simulink model "quadSimulationEnvironment"  (R2022b)
settings: Solver=ode4  StartTime=0.0  StopTime=20  FixedStep=.005  RelTol=1e-3  EnableMultiTasking=on
InitFcn:
  | %%General
  | dT = .005;
  | m = .68;
  | g = 9.8;
  | mg = m*g;
  | 
  | s = tf('s');
  | %%Servomotors
  | h_alpha = 200;
  | 
  | servo_limit = 2500;
  | servo_ratelimit = 450*pi/180/1.33e-4;
  | servo_sampleDelay = 1;
  | servo_wn = 28;
  | servo_zeta = .6;
  | servo_dtime = 5e-3;
  | servo_res = 10;
  | servo_sf = 1/6700;
  | %motor
  | motor_w = 20;
  | motor_dtime = 5e-3;
  | motor_wo = 600;
  | %%Rotors
  | Pw_v = .244/(1+s*.287);
  | Pw_a = -.10/(1+s*.30)*eye(4,4);
  | 
  | motor_limit = 13107;
  | %%Speed control
  | xw = .102/.234;
  | Xw = xw*eye(4,4);
  | 
  | fw = 1/(1+s/1);
  | Fw = fw*eye(4,4);
  | Fw = c2d(Fw,.005,'tustin');
  | 
  | gw = 12.77*(1+s/4)/s/(1+s/21);
  | Gw = gw*eye(4,4);
  | Gw = c2d(Gw,.005,'tustin');
  | %%Thrust control
  | gf = 10628*(1+s/26)*(1+s/44)/s/(1+s/247);
  | Gf = gf*eye(4,4);
  | Gf = c2d(Gf,.005,'tustin');
  | 
  | xf = 358/( s^2/21^2+2*.38/21*s+1);
  | Xf = xf*eye(4,4);
  | Xf = c2d(Xf,.005,'tustin');
  | 
  | %%Attitude control
  | gxy = 7.77*(s+.6443)/(s+268.4);
  | gz = .062*(1+s/3.37)/s/(1+s/169);
  | Gn = [gxy 0 0;
  |       0 gxy 0;
  |       0 0 gz];
  | Gn = c2d(Gn,.005,'tustin');
  | 
  | %%Position control
  | % gp = 151.34*(s+1.925)/(s+81.18);
  | gp = 117.96*(s+0.5)*(s+0.7839)/s/(s+71.75);
  | Gp = gp*eye(3);
  | Gp = c2d(Gp,.005,'tustin');
  | 
  | wp = 4;
  | zp = 1.0;
  | fp = wp^2/(s^2+2*zp*wp*s+wp^2);
  | Fp = fp*eye(3);
  | Fp = c2d(Fp,.005,'tustin');
  | 
  | xp = -.34*(1+s/.5)/(1+s/25.57)*(1+s/11.93)/(1+s/21.7);
  | Xp = xp*eye(3);
  | Xp = c2d(Xp,.005,'tustin');
undefined symbols (not defined in the file or in its folder): Kp, pl_wn, pl_z, w_der, wf_p1, wf_p2, wf_z1, wf_z2, wmr, wp_p, wp_z, wp_z2, wt, zmr, zt
libraries: cstblocks x14, simulink_extras x6, simulink x5, sharedutil x5, uavutilslib x1, matrix_library x1, aerolibutil x1
settings Model: Creator=Arnold  LastModifiedBy=arnoldpretorius
settings SolverCC: AlgebraicLoopSolver=TrustRegion
settings DataIOCC: LimitDataPoints=on  SaveFormat=Array  ReturnWorkspaceOutputs=off
settings OptimizationCC: ExpressionDepthLimit=2147483647  LifeSpan=inf
settings DebuggingCC: UnderspecifiedInitializationDetection=Classic  MergeDetectMultiDrivingBlocksExec=none  SolverPrmCheckMsg=warning  UnconnectedInputMsg=warning  UnconnectedOutputMsg=warning  UnconnectedLineMsg=warning  StateNameClashWarn=warning  SFUnexpectedBacktrackingDiag=warning  SFNoUnconditionalDefaultTransitionDiag=warning  SFExecutionAtInitializationDiag=none  SFMachineParentedDataDiag=warning  ArithmeticOperatorsInVariantConditions=warning
settings HardwareCC: ProdBitPerPointer=32  ProdBitPerSizeT=32  ProdBitPerPtrDiffT=32  ProdLargestAtomicFloat=None  ProdIntDivRoundTo=Undefined  ProdEndianess=Unspecified  ProdWordSize=32  ProdHWDeviceType=32-bit Generic
settings ModelReferenceCC: EnableRefExpFcnMdlSchedulingChecks=on  PropagateSignalLabelsOutOfModel=off
settings SFSimCC: SimUseLocalCustomCode=off  CustomCodeUndefinedFunction=UseInterfaceOnly
settings RTWCC: RTWUseLocalCustomCode=off  DLArmComputeVersion=19.05
settings CodeAppCC: StateflowObjectComments=on
settings GRTTargetCC: TargetLangStandard=C89/C90 (ANSI)
settings ConfigComp: CovMetricSettings=dw  CovSaveCumulativeToWorkspaceVar=on  CovSaveSingleToWorkspaceVar=on  CovExternalEMLEnable=off

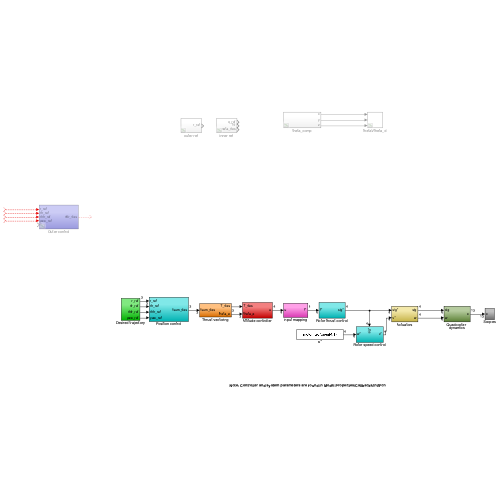
[thumbnail: Simulink's stored preview of the top-level diagram]
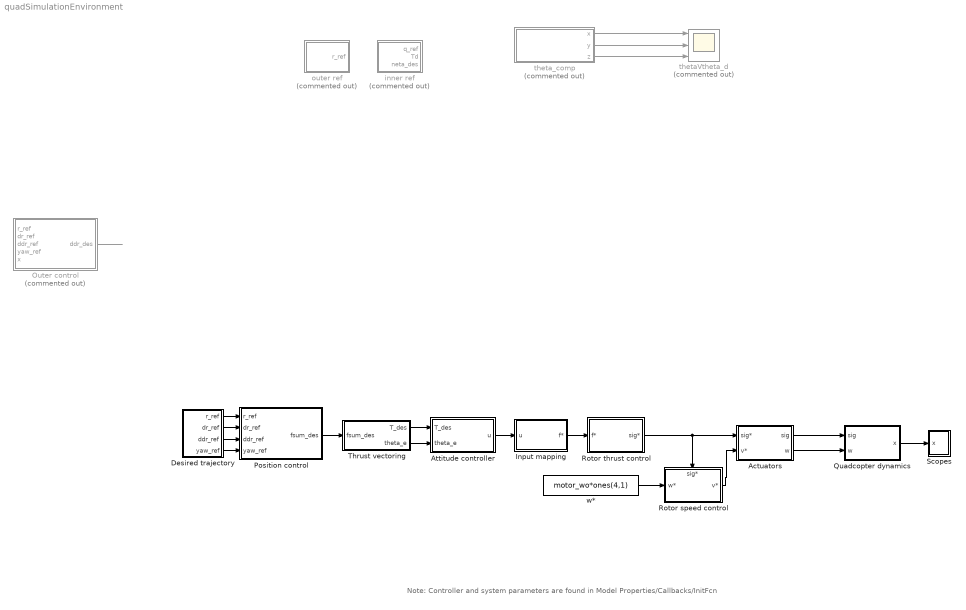
== system quadSimulationEnvironment ==
  note: Note: Controller and system parameters are found in Model Properties/Callbacks/InitFcn
  Actuators : Subsystem
  Attitude controller : Subsystem
  Desired trajectory : Subsystem
  Input mapping : Subsystem
  Outer control : Subsystem  Commented=on
  Position control : Subsystem
  Quadcopter dynamics : Subsystem
  Rotor speed control : Subsystem
      settings: PortSchema="{\"entries\":[{\"content\":{\"sides\":[{\"content\":{\"connectorIds\":[\"In1\"]},\"type\":\"ConnectorPlacement.EquallySpacedRectSide\",\"uuid\":\"a553ec9c-58d4-4b9a-a914-c6161034d4ac\"},{\"content\":{\"connectorIds\":[\"Out1\"],\"side\":\"RIGHT\"},\"type\":\"ConnectorPlacement.EquallySpacedRectSide\",\"uuid\":\"56d1cb9b-318c-4753-8a79-3897c75d4c58\"},{\"content\":{\"connectorIds\":[\"In2\"],\"side\":\"TOP\"},\"type\":\"ConnectorPlacement.EquallySpacedRectSide\",\"uuid\":\"ddf4192e-7ef8-4e19-bd18-fba4d537495f\"}]},\"type\":\"ConnectorPlacement.EquallySpacedConnector\",\"uuid\":\"ae11febd-5c1c-44f7-8744-831945371bf2\"}],\"packageUris\":[\"http://schema.mathworks.com/mf0/Connector/R2020b\"],\"version\":\"1.0\"}"
  Rotor thrust control : Subsystem
  Scopes : Subsystem
  Thrust vectoring : Subsystem
  inner ref : Subsystem  Commented=on
  outer ref : Subsystem  Commented=on
  thetaVtheta_d : Scope  Commented=on  NumInputPorts=3
  theta_comp : Subsystem  Commented=on
  w* : Constant  Value=motor_wo*ones(4,1)
  wires:
  Quadcopter dynamics/1(x) -> Scopes/1(x)
  Outer control/1(ddr_des) -> ?
  Actuators/1(sig) -> Quadcopter dynamics/1(sig)
  Actuators/2(w) -> Quadcopter dynamics/2(w)
  ? -> Outer control/1(r_ref)
  ? -> Outer control/2(dr_ref)
  ? -> Outer control/3(ddr_ref)
  ? -> Outer control/4(yaw_ref)
  Rotor thrust control/1(sig*) -> Actuators/1(sig*), Rotor speed control/2(sig*)
  Rotor speed control/1(v*) -> Actuators/2(v*)
  Input mapping/1(f*) -> Rotor thrust control/1(f*)
  Attitude controller/1(u) -> Input mapping/1(u)
  Thrust vectoring/1(T_des) -> Attitude controller/1(T_des)
  Thrust vectoring/2(theta_e) -> Attitude controller/2(theta_e)
  theta_comp/1(x) -> thetaVtheta_d/1
  theta_comp/3(z) -> thetaVtheta_d/3
  theta_comp/2(y) -> thetaVtheta_d/2
  Position control/1(fsum_des) -> Thrust vectoring/1(fsum_des)
  Desired trajectory/2(dr_ref) -> Position control/2(dr_ref)
  Desired trajectory/4(yaw_ref) -> Position control/4(yaw_ref)
  Desired trajectory/1(r_ref) -> Position control/1(r_ref)
  Desired trajectory/3(ddr_ref) -> Position control/3(ddr_ref)
  w*/1 -> Rotor speed control/1(w*)

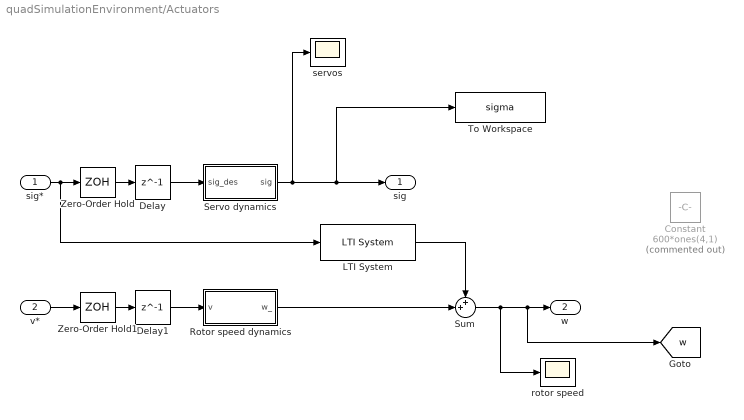
== system quadSimulationEnvironment/Actuators ==
  sig* : Inport
  v* : Inport  Port=2
  Constant : Constant  Commented=on  Value=600*ones(4,1)
  Delay : Delay  DelayLength=1  SampleTime=dT
  Delay1 : Delay  DelayLength=1  SampleTime=dT
  LTI System : cstblocks/LTI System  sys=Pw_a  IC=[]
  Rotor speed dynamics : Subsystem
  Servo dynamics : Subsystem
  Sum : Sum  Inputs=++|
  To Workspace : ToWorkspace  VariableName=sigma  SaveFormat=Timeseries  SampleTime=-1
  Zero-Order Hold : ZeroOrderHold  SampleTime=servo_dtime
  Zero-Order Hold1 : ZeroOrderHold  SampleTime=motor_dtime
  rotor speed : Scope
  servos : Scope
  sig : Outport
  w : Outport  Port=2
  tag scope: w=global
  wires:
  Servo dynamics/1(sig) -> servos/1, To Workspace/1, sig/1
  sig*/1 -> LTI System/1, Zero-Order Hold/1
  v*/1 -> Zero-Order Hold1/1
  Delay1/1 -> Rotor speed dynamics/1(v)
  Delay/1 -> Servo dynamics/1(sig_des)
  Zero-Order Hold/1 -> Delay/1
  Zero-Order Hold1/1 -> Delay1/1
  Sum/1 -> rotor speed/1, [w], w/1
  Rotor speed dynamics/1(w_) -> Sum/2
  LTI System/1 -> Sum/1

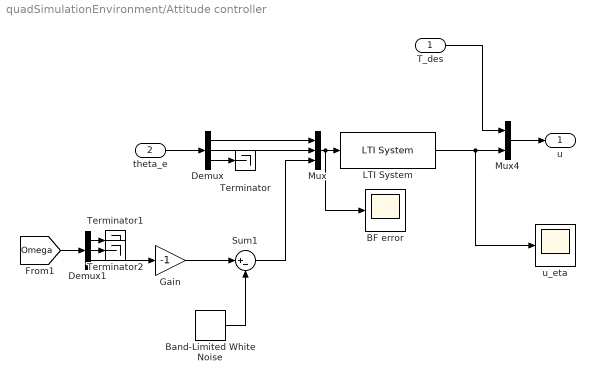
== system quadSimulationEnvironment/Attitude controller ==
  T_des : Inport
  theta_e : Inport  Port=2
  BF error : Scope
  Band-Limited White Noise : simulink/Sources/Band-Limited White Noise  Cov=[0.0004]  Ts=0.005  seed=[123]
  Demux : Demux  Outputs=3
  Demux1 : Demux  Outputs=3
  Gain : Gain  Gain=-1
  LTI System : cstblocks/LTI System  sys=Gn  IC=[]
  Mux : Mux  Inputs=3
  Mux4 : Mux  Inputs=2
  Sum1 : Sum  Inputs=|+-
  Terminator : Terminator
  Terminator1 : Terminator
  Terminator2 : Terminator
  u_eta : Scope
  u : Outport
  wires:
  LTI System/1 -> u_eta/1, Mux4/2
  Mux4/1 -> u/1
  T_des/1 -> Mux4/1
  theta_e/1 -> Demux/1
  Mux/1 -> BF error/1, LTI System/1
  Demux/1 -> Mux/1
  Demux/2 -> Mux/2
  Demux/3 -> Terminator/1
  [Omega] -> Demux1/1
  Demux1/3 -> Gain/1
  Demux1/1 -> Terminator1/1
  Demux1/2 -> Terminator2/1
  Gain/1 -> Sum1/1
  Sum1/1 -> Mux/3
  Band-Limited White Noise/1 -> Sum1/2

== system quadSimulationEnvironment/Desired trajectory ==
  Gain : Gain  Gain=-1
  LTI System : cstblocks/LTI System  sys=fp  IC=[]
  LTI System1 : cstblocks/LTI System  sys=fp  IC=[]
  Mux1 : Mux  Inputs=3
  Step1 : Step  Time=10  SampleTime=0
  Step2 : Step  Time=3  SampleTime=0
  r_ref : Outport
  dr_ref : Outport  Port=2
  ddr_ref : Outport  Port=3
  yaw_ref : Outport  Port=4
  wires:
  Mux1/1 -> r_ref/1
  Step1/1 -> LTI System/1
  Gain/1 -> Mux1/2
  Step2/1 -> LTI System1/1
  LTI System/1 -> Gain/1, Mux1/1
  LTI System1/1 -> Mux1/3

== system quadSimulationEnvironment/Input mapping ==
  u : Inport
  Display1 : Display
  Display2 : Display
  "input2sig_des " : MATLAB Function  TreatAsAtomicUnit=on
  mixing : MATLAB Function  Commented=on  TreatAsAtomicUnit=on
  yawFreeSig : MATLAB Function  Commented=on  TreatAsAtomicUnit=on
  f* : Outport
  wires:
  u/1 -> "input2sig_des "/1(u)
  "input2sig_des "/1(f_des) -> Display1/1, f*/1

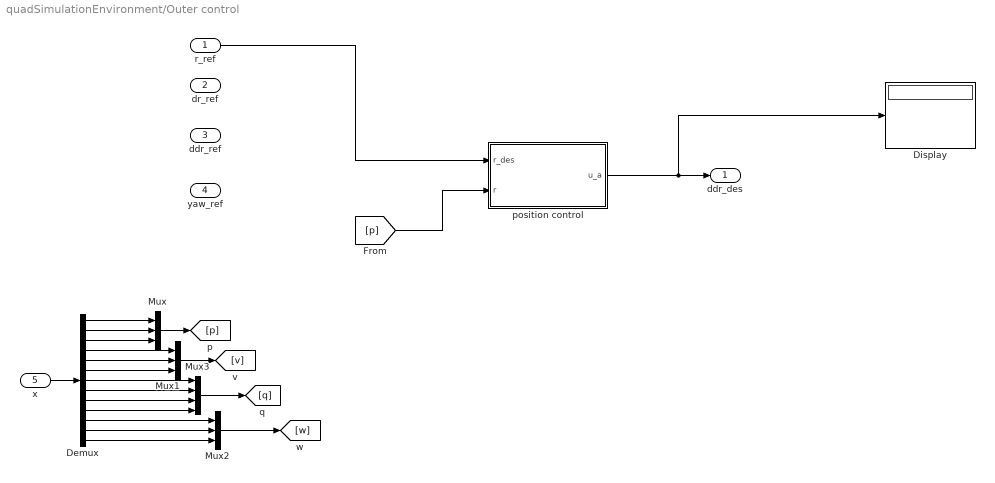
== system quadSimulationEnvironment/Outer control ==
  r_ref : Inport
  dr_ref : Inport  Port=2
  ddr_ref : Inport  Port=3
  yaw_ref : Inport  Port=4
  x : Inport  Port=5
  Demux : Demux  Outputs=13
  Display : Display
  Mux : Mux  Inputs=3
  Mux1 : Mux  Inputs=3
  Mux2 : Mux  Inputs=3
  Mux3 : Mux
  position control : Subsystem
  ddr_des : Outport
  wires:
  r_ref/1 -> position control/1(r_des)
  [p] -> position control/2(r)
  position control/1(u_a) -> Display/1, ddr_des/1
  x/1 -> Demux/1
  Demux/1 -> Mux/1
  Demux/2 -> Mux/2
  Demux/3 -> Mux/3
  Demux/4 -> Mux1/1
  Demux/5 -> Mux1/2
  Demux/6 -> Mux1/3
  Demux/7 -> Mux3/1
  Demux/8 -> Mux3/2
  Demux/9 -> Mux3/3
  Mux1/1 -> [v]
  Mux/1 -> [p]
  Demux/10 -> Mux3/4
  Demux/11 -> Mux2/1
  Demux/12 -> Mux2/2
  Demux/13 -> Mux2/3
  Mux3/1 -> [q]
  Mux2/1 -> [w]

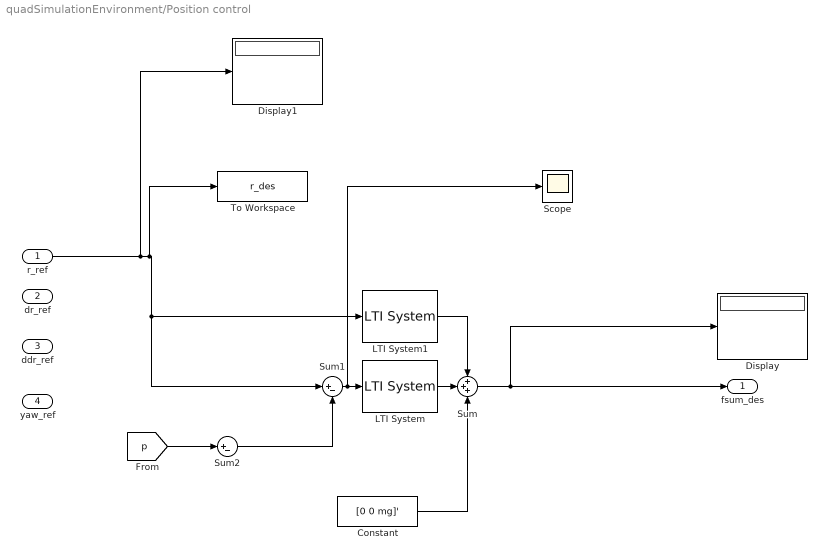
== system quadSimulationEnvironment/Position control ==
  r_ref : Inport
  dr_ref : Inport  Port=2
  ddr_ref : Inport  Port=3
  yaw_ref : Inport  Port=4
  Constant : Constant  Value=[0 0 mg]'
  Display : Display
  Display1 : Display
  LTI System : cstblocks/LTI System  sys=Gp  IC=[]
  LTI System1 : cstblocks/LTI System  sys=Xp  IC=[]
  Scope : Scope
  Sum : Sum  Inputs=+++
  Sum1 : Sum  Inputs=|+-
  Sum2 : Sum  Inputs=|+-
  To Workspace : ToWorkspace  VariableName=r_des  SaveFormat=Timeseries  SampleTime=-1
  fsum_des : Outport
  wires:
  r_ref/1 -> Display1/1, To Workspace/1, LTI System1/1, Sum1/1
  Sum/1 -> Display/1, fsum_des/1
  LTI System/1 -> Sum/2
  Constant/1 -> Sum/3
  Sum1/1 -> Scope/1, LTI System/1
  [p] -> Sum2/1
  Sum2/1 -> Sum1/2
  LTI System1/1 -> Sum/1

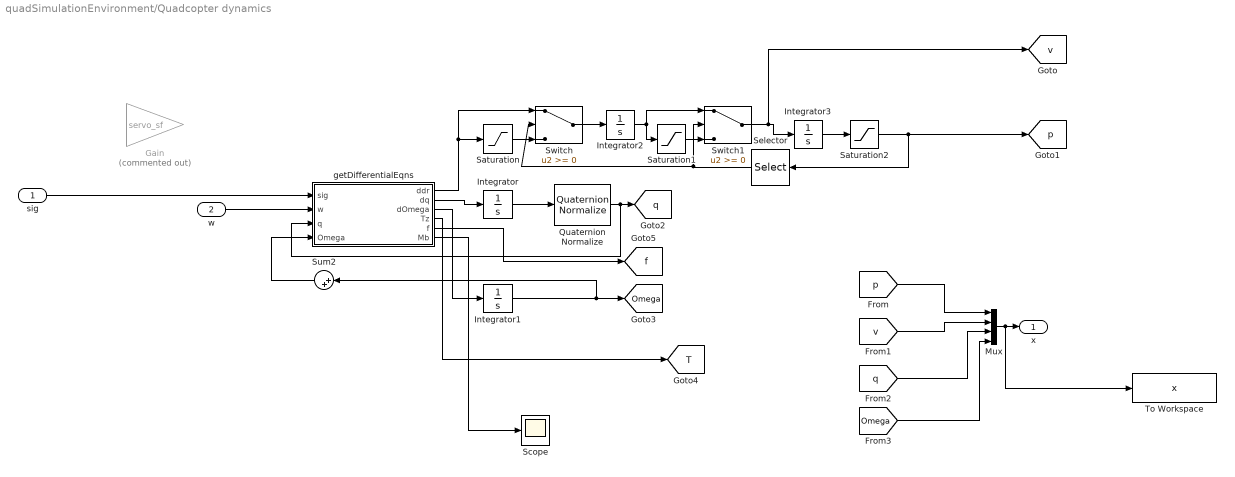
== system quadSimulationEnvironment/Quadcopter dynamics ==
  sig : Inport
  w : Inport  Port=2
  Gain : Gain  Commented=on  Gain=servo_sf
  Integrator : Integrator  InitialCondition=[1 0 0 0]
  Integrator1 : Integrator  InitialCondition=[0 0 0]
  Integrator2 : Integrator  InitialCondition=[0 0 0]
  Integrator3 : Integrator  InitialCondition=[0 0 0]
  Mux : Mux
  Quaternion Normalize : sharedutil/Quaternion Normalize  aMode=aMode
  Saturation : Saturate  UpperLimit=[1e10 1e10 1e10]  LowerLimit=[-1e10 -1e10 0]
  Saturation1 : Saturate  UpperLimit=[1e10 1e10 1e10]  LowerLimit=[-1e10 -1e10 0]
  Saturation2 : Saturate  UpperLimit=[1e10 1e10 1e10]  LowerLimit=[-1e10 -1e10 0]
  Scope : Scope
  Selector : Selector  InputPortWidth=3  IndexOptions=Index vector (dialog)  Indices=[3]  OutputSizes=1
  Sum2 : Sum  Inputs=|++
  Switch : Switch  SaturateOnIntegerOverflow=off  InputSameDT=off
  Switch1 : Switch  SaturateOnIntegerOverflow=off  InputSameDT=off
  To Workspace : ToWorkspace  VariableName=x  SaveFormat=Timeseries  SampleTime=-1
  getDifferentialEqns : MATLAB Function  TreatAsAtomicUnit=on
  x : Outport
  tag scope: Omega=global, T=global, f=global, p=global, q=global, v=global
  wires:
  w/1 -> getDifferentialEqns/2(w)
  getDifferentialEqns/2(dq) -> Integrator/1
  Integrator/1 -> Quaternion Normalize/1
  getDifferentialEqns/3(dOmega) -> Integrator1/1
  Integrator1/1 -> Sum2/1, [Omega]
  Integrator3/1 -> Saturation2/1
  Mux/1 -> To Workspace/1, x/1
  [p] -> Mux/1
  [v] -> Mux/2
  [q] -> Mux/3
  [Omega] -> Mux/4
  getDifferentialEqns/4(Tz) -> [T]
  getDifferentialEqns/5(f) -> [f]
  sig/1 -> getDifferentialEqns/1(sig)
  Quaternion Normalize/1 -> getDifferentialEqns/3(q), [q]
  getDifferentialEqns/6(Mb) -> Scope/1
  getDifferentialEqns/1(ddr) -> Saturation/1, Switch/1
  Sum2/1 -> getDifferentialEqns/4(Omega)
  Saturation/1 -> Switch/3
  Switch/1 -> Integrator2/1
  Integrator2/1 -> Saturation1/1, Switch1/1
  Saturation1/1 -> Switch1/3
  Switch1/1 -> [v], Integrator3/1
  Saturation2/1 -> Selector/1, [p]
  Selector/1 -> Switch1/2, Switch/2

== system quadSimulationEnvironment/Rotor speed control ==
  w* : Inport
  sig* : Inport  Port=2
  LTI System : cstblocks/LTI System  sys=Gw  IC=[]
  LTI System1 : cstblocks/LTI System  sys=Xw  IC=[]
  Sum : Sum  Inputs=|+-
  Sum1 : Sum  Inputs=++|
  v* : Outport
  wires:
  w*/1 -> Sum/1
  [w] -> Sum/2
  Sum/1 -> LTI System/1
  LTI System/1 -> Sum1/2
  LTI System1/1 -> Sum1/1
  Sum1/1 -> v*/1
  sig*/1 -> LTI System1/1

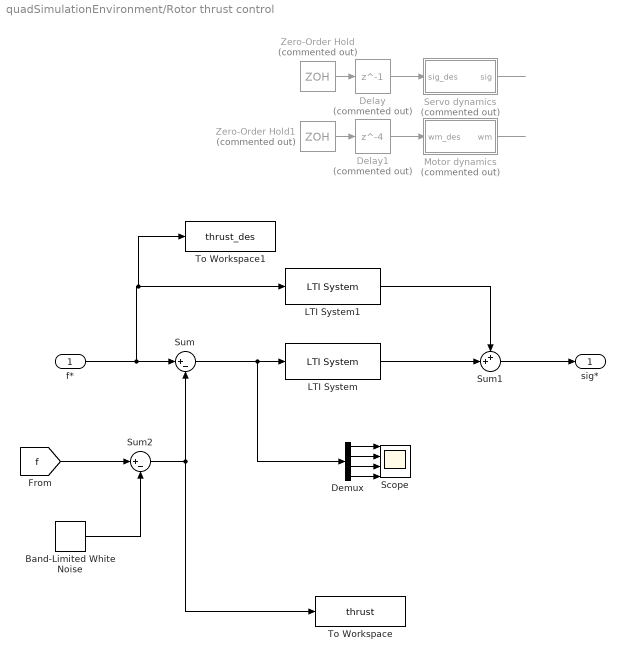
== system quadSimulationEnvironment/Rotor thrust control ==
  f* : Inport
  Band-Limited White Noise : simulink/Sources/Band-Limited White Noise  Cov=[0.000008]  Ts=0.005  seed=[23341]
  Delay : Delay  Commented=on  DelayLength=1  SampleTime=dT
  Delay1 : Delay  Commented=on  DelayLength=4  SampleTime=dT
  Demux : Demux
  LTI System : cstblocks/LTI System  sys=Gf  IC=[]
  LTI System1 : cstblocks/LTI System  sys=Xf  IC=[]
  Motor dynamics : Subsystem  Commented=on
  Scope : Scope  NumInputPorts=4
  Servo dynamics : Subsystem  Commented=on
  Sum : Sum  Inputs=|+-
  Sum1 : Sum  Inputs=++|
  Sum2 : Sum  Inputs=|+-
  To Workspace : ToWorkspace  VariableName=thrust  SaveFormat=Timeseries  SampleTime=-1
  To Workspace1 : ToWorkspace  VariableName=thrust_des  SaveFormat=Timeseries  SampleTime=-1
  Zero-Order Hold : ZeroOrderHold  Commented=on  SampleTime=servo_dtime
  Zero-Order Hold1 : ZeroOrderHold  Commented=on  SampleTime=motor_dtime
  sig* : Outport
  wires:
  Delay1/1 -> Motor dynamics/1(wm_des)
  Zero-Order Hold/1 -> Delay/1
  Zero-Order Hold1/1 -> Delay1/1
  Delay/1 -> Servo dynamics/1(sig_des)
  Motor dynamics/1(wm) -> ?
  Servo dynamics/1(sig) -> ?
  f*/1 -> To Workspace1/1, LTI System1/1, Sum/1
  Sum1/1 -> sig*/1
  [f] -> Sum2/1
  Sum/1 -> Demux/1, LTI System/1
  LTI System1/1 -> Sum1/1
  LTI System/1 -> Sum1/2
  Demux/1 -> Scope/1
  Demux/2 -> Scope/2
  Demux/3 -> Scope/3
  Demux/4 -> Scope/4
  Sum2/1 -> To Workspace/1, Sum/2
  Band-Limited White Noise/1 -> Sum2/2

== system quadSimulationEnvironment/Scopes ==
  x : Inport
  .1 : MATLAB Function  TreatAsAtomicUnit=on
  Omega : Scope
  Radians to Degrees : simulink_extras/Transformations/Radians to Degrees
  Radians to Degrees1 : simulink_extras/Transformations/Radians to Degrees
  UAV Animation : uavutilslib/UAV Animation  UAVType=Multirotor  UAVSize=1  InertialZDirection=Up  SampleTime=-1
  dr : Scope
  eta : Scope
  q : Scope
  r : Scope
  wires:
  x/1 -> .1/1(x)
  .1/1(R_i) -> r/1
  .1/2(dR_i) -> dr/1
  .1/3(Omega_b) -> Radians to Degrees1/1
  .1/5(q) -> q/1
  .1/4(eta) -> Radians to Degrees/1
  Radians to Degrees/1 -> eta/1
  Radians to Degrees1/1 -> Omega/1
  [p] -> UAV Animation/1
  [q] -> UAV Animation/2

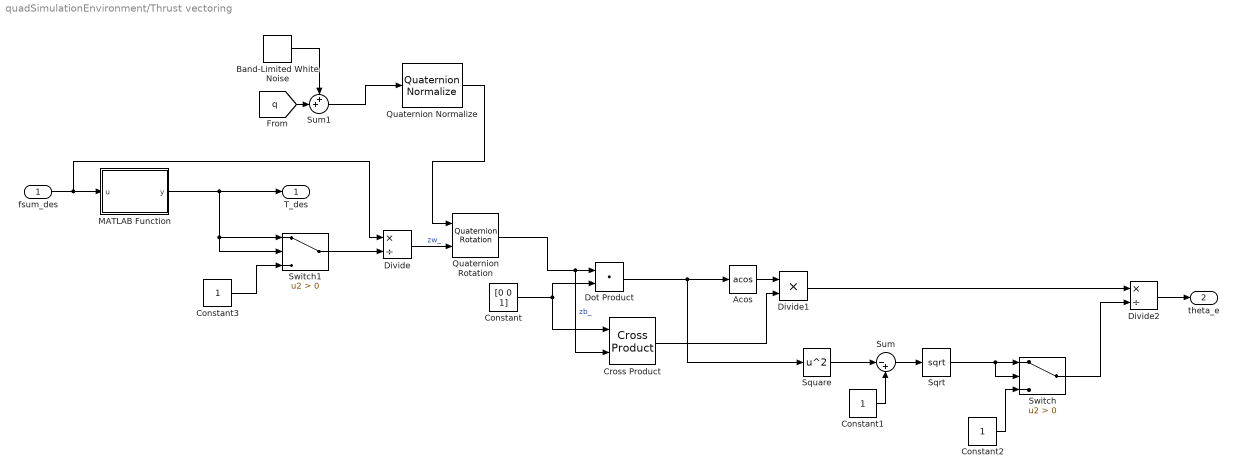
== system quadSimulationEnvironment/Thrust vectoring ==
  fsum_des : Inport
  Acos : Trigonometry  Operator=acos
  Band-Limited White Noise : simulink/Sources/Band-Limited White Noise  Cov=[0.000001]  Ts=0.005  seed=[233141]
  Constant : Constant  Value=[0 0 1]
  Constant1 : Constant
  Constant2 : Constant
  Constant3 : Constant
  Cross Product : matrix_library/Cross Product
  Divide : Product  Inputs=*/
  Divide1 : Product  Inputs=**
  Divide2 : Product  Inputs=*/
  Dot Product : DotProduct  OutDataTypeStr=Inherit: Inherit via internal rule
  MATLAB Function : MATLAB Function  TreatAsAtomicUnit=on
  Quaternion Normalize : sharedutil/Quaternion Normalize  aMode=aMode
  Quaternion Rotation : aerolibutil/Quaternion Rotation
  Sqrt : Sqrt
  Square : Math  Operator=square
  Sum : Sum  Inputs=|-+
  Sum1 : Sum  Inputs=++|
  Switch : Switch  Criteria=u2 > Threshold  SaturateOnIntegerOverflow=off  InputSameDT=off
  Switch1 : Switch  Criteria=u2 > Threshold  SaturateOnIntegerOverflow=off  InputSameDT=off
  T_des : Outport
  theta_e : Outport  Port=2
  wires:
  fsum_des/1 -> MATLAB Function/1(u), Divide/1
  Divide2/1 -> theta_e/1
  MATLAB Function/1(y) -> Switch1/2, Switch1/1, T_des/1
  Constant/1 -> Cross Product/1, Dot Product/2
  Dot Product/1 -> Square/1, Acos/1
  Acos/1 -> Divide1/1
  Cross Product/1 -> Divide1/2
  Divide1/1 -> Divide2/1
  Sum/1 -> Sqrt/1
  Constant1/1 -> Sum/2
  Square/1 -> Sum/1
  Divide/1 -> Quaternion Rotation/2  "zw_"
  Quaternion Rotation/1 -> Cross Product/2, Dot Product/1  "zb_"
  Sqrt/1 -> Switch/2, Switch/1
  Switch/1 -> Divide2/2
  Constant2/1 -> Switch/3
  Switch1/1 -> Divide/2
  Constant3/1 -> Switch1/3
  Quaternion Normalize/1 -> Quaternion Rotation/1
  [q] -> Sum1/2
  Band-Limited White Noise/1 -> Sum1/1
  Sum1/1 -> Quaternion Normalize/1

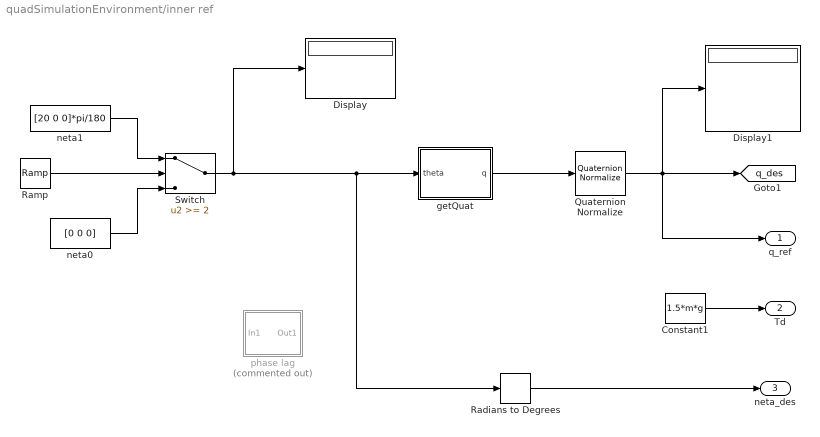
== system quadSimulationEnvironment/inner ref ==
  Constant1 : Constant  Value=1.5*m*g
  Display : Display
  Display1 : Display
  Quaternion Normalize : sharedutil/Quaternion Normalize  aMode=aMode
  Radians to Degrees : simulink_extras/Transformations/Radians to Degrees
  Ramp : simulink/Sources/Ramp  slope=1  start=0  InitialOutput=0
  Switch : Switch  Threshold=2  SaturateOnIntegerOverflow=off  InputSameDT=off
  getQuat : MATLAB Function  TreatAsAtomicUnit=on
  neta0 : Constant  Value=[0 0 0]
  neta1 : Constant  Value=[20 0 0]*pi/180
  phase lag : Subsystem  Commented=on
  q_ref : Outport
  Td : Outport  Port=2
  neta_des : Outport  Port=3
  tag scope: q_des=global
  wires:
  Constant1/1 -> Td/1
  neta1/1 -> Switch/1
  Ramp/1 -> Switch/2
  neta0/1 -> Switch/3
  getQuat/1(q) -> Quaternion Normalize/1
  Radians to Degrees/1 -> neta_des/1
  Switch/1 -> getQuat/1(theta), Radians to Degrees/1, Display/1
  Quaternion Normalize/1 -> q_ref/1, [q_des], Display1/1

== system quadSimulationEnvironment/outer ref ==
  Display : Display
  Ramp : simulink/Sources/Ramp  slope=1  start=0  X0=0
  Switch : Switch  Threshold=5  SaturateOnIntegerOverflow=off  InputSameDT=off
  phase lag : Subsystem
  r_des : Constant  Commented=on  Value=[0 0 .3]
  r_des0 : Constant  Value=[0 0 0]
  r_des1 : Constant  Value=[1 0 0]
  r_ref : Outport
  wires:
  phase lag/1(Out1) -> r_ref/1
  r_des1/1 -> Switch/1
  Ramp/1 -> Switch/2
  r_des0/1 -> Switch/3
  Switch/1 -> phase lag/1(In1), Display/1

== system quadSimulationEnvironment/theta_comp ==
  3vec_comp : Subsystem
  Quaternion Normalize : sharedutil/Quaternion Normalize  aMode=aMode
  Quaternion Normalize1 : sharedutil/Quaternion Normalize  aMode=aMode
  Radians to Degrees : simulink_extras/Transformations/Radians to Degrees
  Radians to Degrees1 : simulink_extras/Transformations/Radians to Degrees
  Radians to Degrees2 : simulink_extras/Transformations/Radians to Degrees
  getRotVec : MATLAB Function  TreatAsAtomicUnit=on
  getRotVec1 : MATLAB Function  TreatAsAtomicUnit=on
  x : Outport
  y : Outport  Port=2
  z : Outport  Port=3
  wires:
  [q] -> Quaternion Normalize/1
  [q_des] -> Quaternion Normalize1/1
  getRotVec1/1(theta) -> 3vec_comp/1(des)
  getRotVec/1(theta) -> 3vec_comp/2(meas)
  3vec_comp/1(comp_x) -> Radians to Degrees/1
  3vec_comp/2(comp_y) -> Radians to Degrees1/1
  3vec_comp/3(comp_z) -> Radians to Degrees2/1
  Quaternion Normalize/1 -> getRotVec/1(q)
  Quaternion Normalize1/1 -> getRotVec1/1(q)
  Radians to Degrees/1 -> x/1
  Radians to Degrees1/1 -> y/1
  Radians to Degrees2/1 -> z/1

== system quadSimulationEnvironment/Actuators/Rotor speed dynamics ==
  v : Inport
  Demux10 : Demux
  Display : Display
  LTI System{,1..3} (4 alike) : cstblocks/LTI System  sys=Pw_v  IC=[]
  Mux4 : Mux
  Saturation{1..4} (4 alike) : Saturate  UpperLimit=motor_limit  LowerLimit=0
  Transfer Fcn : TransferFcn  Commented=on  Numerator=[-.008/2 1]  Denominator=[.008/2 1]
  u : Scope
  w_ : Outport
  wires:
  v/1 -> Display/1, Demux10/1
  Demux10/1 -> Saturation4/1
  Mux4/1 -> u/1, w_/1
  LTI System/1 -> Mux4/1
  Saturation4/1 -> LTI System/1
  Demux10/2 -> Saturation1/1
  Saturation1/1 -> LTI System1/1
  LTI System1/1 -> Mux4/2
  Demux10/3 -> Saturation2/1
  Saturation2/1 -> LTI System2/1
  Demux10/4 -> Saturation3/1
  Saturation3/1 -> LTI System3/1
  LTI System2/1 -> Mux4/3
  LTI System3/1 -> Mux4/4

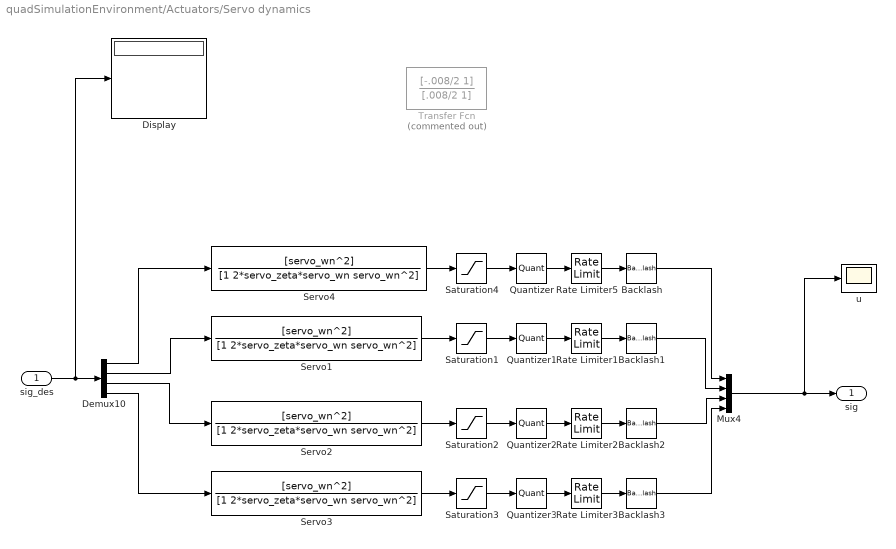
== system quadSimulationEnvironment/Actuators/Servo dynamics ==
  sig_des : Inport
  Backlash{,1..3} (4 alike) : Backlash  BacklashWidth=h_alpha
  Demux10 : Demux
  Display : Display
  Mux4 : Mux
  Quantizer{,1..3} (4 alike) : Quantizer  QuantizationInterval=servo_res
  Rate Limiter{1..3,5} (4 alike) : RateLimiter  RisingSlewLimit=servo_ratelimit  FallingSlewLimit=-servo_ratelimit  SampleTimeMode=inherited
  Saturation{1..4} (4 alike) : Saturate  UpperLimit=servo_limit  LowerLimit=-servo_limit
  Servo{1..4} (4 alike) : TransferFcn  Numerator=[servo_wn^2]  Denominator=[1 2*servo_zeta*servo_wn servo_wn^2]
  Transfer Fcn : TransferFcn  Commented=on  Numerator=[-.008/2 1]  Denominator=[.008/2 1]
  u : Scope
  sig : Outport
  wires:
  Demux10/3 -> Servo2/1
  sig_des/1 -> Display/1, Demux10/1
  Demux10/1 -> Servo4/1
  Demux10/2 -> Servo1/1
  Demux10/4 -> Servo3/1
  Saturation4/1 -> Quantizer/1
  Saturation1/1 -> Quantizer1/1
  Saturation2/1 -> Quantizer2/1
  Saturation3/1 -> Quantizer3/1
  Mux4/1 -> u/1, sig/1
  Servo4/1 -> Saturation4/1
  Servo1/1 -> Saturation1/1
  Servo2/1 -> Saturation2/1
  Servo3/1 -> Saturation3/1
  Quantizer/1 -> Rate Limiter5/1
  Quantizer1/1 -> Rate Limiter1/1
  Quantizer2/1 -> Rate Limiter2/1
  Quantizer3/1 -> Rate Limiter3/1
  Rate Limiter5/1 -> Backlash/1
  Rate Limiter1/1 -> Backlash1/1
  Rate Limiter2/1 -> Backlash2/1
  Rate Limiter3/1 -> Backlash3/1
  Backlash/1 -> Mux4/1
  Backlash1/1 -> Mux4/2
  Backlash2/1 -> Mux4/3
  Backlash3/1 -> Mux4/4

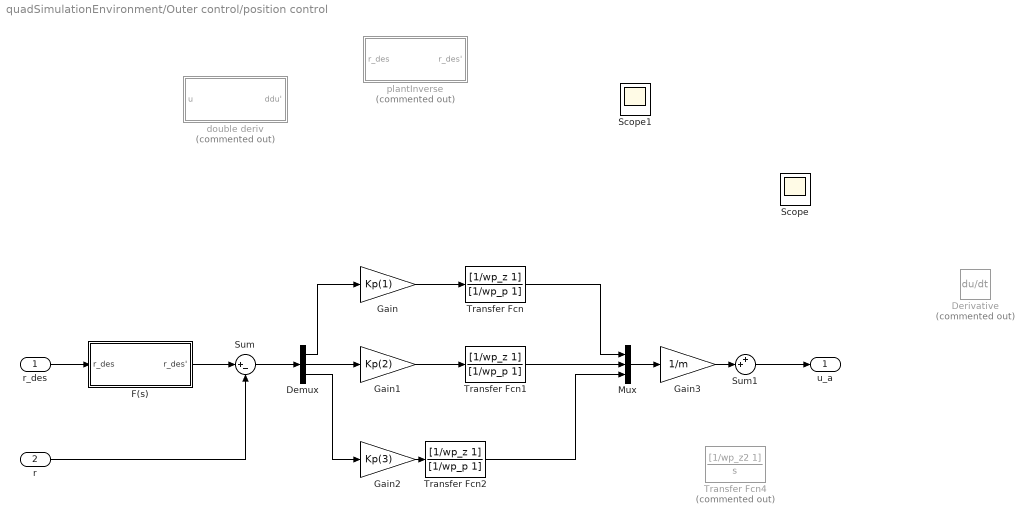
== system quadSimulationEnvironment/Outer control/position control ==
  r_des : Inport
  r : Inport  Port=2
  Demux : Demux  Outputs=3
  Derivative : Derivative  Commented=on  CoefficientInTFapproximation=1/100
  F(s) : Subsystem
  Gain : Gain  Gain=Kp(1)
  Gain1 : Gain  Gain=Kp(2)
  Gain2 : Gain  Gain=Kp(3)
  Gain3 : Gain  Gain=1/m
  Mux : Mux  Inputs=3
  Scope : Scope
  Scope1 : Scope
  Sum : Sum  Inputs=|+-
  Sum1 : Sum  Inputs=++|
  Transfer Fcn : TransferFcn  Numerator=[1/wp_z 1]  Denominator=[1/wp_p 1]
  Transfer Fcn1 : TransferFcn  Numerator=[1/wp_z 1]  Denominator=[1/wp_p 1]
  Transfer Fcn2 : TransferFcn  Numerator=[1/wp_z 1]  Denominator=[1/wp_p 1]
  Transfer Fcn4 : TransferFcn  Commented=on  Numerator=[1/wp_z2 1]  Denominator=[1 0]
  double deriv : Subsystem  Commented=on
  plantInverse : Subsystem  Commented=on
  u_a : Outport
  wires:
  r/1 -> Sum/2
  Mux/1 -> Gain3/1
  Sum/1 -> Demux/1
  Demux/1 -> Gain/1
  Transfer Fcn/1 -> Mux/1
  Demux/2 -> Gain1/1
  Transfer Fcn1/1 -> Mux/2
  Gain/1 -> Transfer Fcn/1
  Gain1/1 -> Transfer Fcn1/1
  Gain2/1 -> Transfer Fcn2/1
  Sum1/1 -> u_a/1
  r_des/1 -> F(s)/1(r_des)
  Gain3/1 -> Sum1/2
  F(s)/1(r_des') -> Sum/1
  Demux/3 -> Gain2/1
  Transfer Fcn2/1 -> Mux/3

== system quadSimulationEnvironment/Rotor thrust control/Motor dynamics ==
  wm_des : Inport
  Demux10 : Demux  Outputs=2
  Mux4 : Mux  Inputs=2
  Sum : Sum  Inputs=++|
  Sum1 : Sum  Inputs=++|
  Transfer Fcn1 : TransferFcn  Denominator=[1/motor_w 1]
  Transfer Fcn2 : TransferFcn  Denominator=[1/motor_w 1]
  wm : Outport
  wires:
  Mux4/1 -> wm/1
  wm_des/1 -> Demux10/1
  Demux10/1 -> Transfer Fcn1/1
  Demux10/2 -> Transfer Fcn2/1
  Sum/1 -> Mux4/1
  Sum1/1 -> Mux4/2
  Transfer Fcn1/1 -> Sum/2
  Transfer Fcn2/1 -> Sum1/2

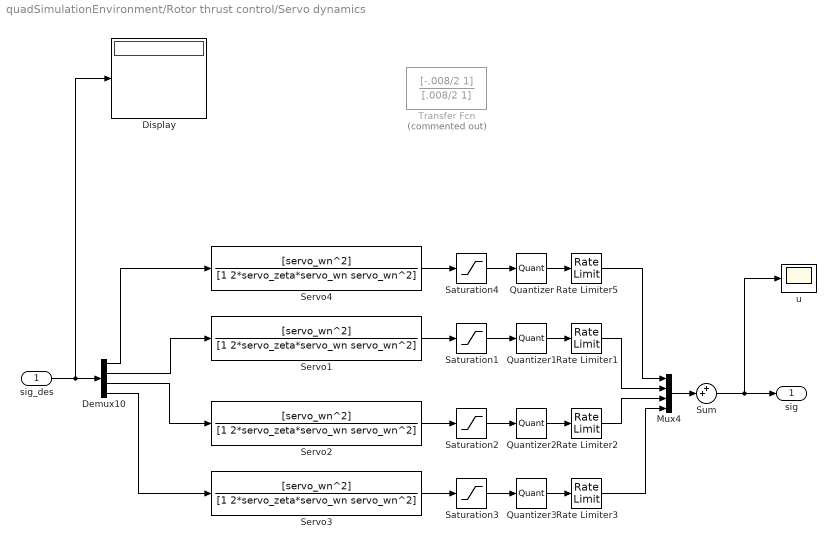
== system quadSimulationEnvironment/Rotor thrust control/Servo dynamics ==
  sig_des : Inport
  Demux10 : Demux
  Display : Display
  Mux4 : Mux
  Quantizer{,1..3} (4 alike) : Quantizer  QuantizationInterval=servo_res
  Rate Limiter{1..3,5} (4 alike) : RateLimiter  RisingSlewLimit=servo_ratelimit  FallingSlewLimit=-servo_ratelimit  SampleTimeMode=inherited
  Saturation{1..4} (4 alike) : Saturate  UpperLimit=servo_limit  LowerLimit=-servo_limit
  Servo{1..4} (4 alike) : TransferFcn  Numerator=[servo_wn^2]  Denominator=[1 2*servo_zeta*servo_wn servo_wn^2]
  Sum : Sum  Inputs=++|
  Transfer Fcn : TransferFcn  Commented=on  Numerator=[-.008/2 1]  Denominator=[.008/2 1]
  u : Scope
  sig : Outport
  wires:
  Demux10/3 -> Servo2/1
  sig_des/1 -> Display/1, Demux10/1
  Demux10/1 -> Servo4/1
  Demux10/2 -> Servo1/1
  Demux10/4 -> Servo3/1
  Saturation4/1 -> Quantizer/1
  Saturation1/1 -> Quantizer1/1
  Saturation2/1 -> Quantizer2/1
  Saturation3/1 -> Quantizer3/1
  Sum/1 -> u/1, sig/1
  Mux4/1 -> Sum/2
  Servo4/1 -> Saturation4/1
  Servo1/1 -> Saturation1/1
  Servo2/1 -> Saturation2/1
  Servo3/1 -> Saturation3/1
  Quantizer/1 -> Rate Limiter5/1
  Quantizer1/1 -> Rate Limiter1/1
  Quantizer2/1 -> Rate Limiter2/1
  Quantizer3/1 -> Rate Limiter3/1
  Rate Limiter5/1 -> Mux4/1
  Rate Limiter1/1 -> Mux4/2
  Rate Limiter2/1 -> Mux4/3
  Rate Limiter3/1 -> Mux4/4

== system quadSimulationEnvironment/inner ref/phase lag ==
  In1 : Inport
  Demux : Demux  Outputs=3
  Mux : Mux  Inputs=3
  Transfer Fcn1 : TransferFcn  Numerator=[pl_wn^2]  Denominator=[1 2*pl_z*pl_wn pl_wn^2]
  Transfer Fcn2 : TransferFcn  Numerator=[pl_wn^2]  Denominator=[1 2*pl_z*pl_wn pl_wn^2]
  Transfer Fcn3 : TransferFcn  Numerator=[pl_wn^2]  Denominator=[1 2*pl_z*pl_wn pl_wn^2]
  Out1 : Outport
  wires:
  Mux/1 -> Out1/1
  In1/1 -> Demux/1
  Demux/1 -> Transfer Fcn3/1
  Demux/2 -> Transfer Fcn1/1
  Demux/3 -> Transfer Fcn2/1
  Transfer Fcn3/1 -> Mux/1
  Transfer Fcn1/1 -> Mux/2
  Transfer Fcn2/1 -> Mux/3

== system quadSimulationEnvironment/outer ref/phase lag ==
  In1 : Inport
  Demux : Demux  Outputs=3
  Mux : Mux  Inputs=3
  Transfer Fcn1 : TransferFcn  Numerator=[pl_wn^2]  Denominator=[1 2*pl_z*pl_wn pl_wn^2]
  Transfer Fcn2 : TransferFcn  Numerator=[pl_wn^2]  Denominator=[1 2*pl_z*pl_wn pl_wn^2]
  Transfer Fcn3 : TransferFcn  Numerator=[pl_wn^2]  Denominator=[1 2*pl_z*pl_wn pl_wn^2]
  Out1 : Outport
  wires:
  Mux/1 -> Out1/1
  In1/1 -> Demux/1
  Demux/1 -> Transfer Fcn3/1
  Demux/2 -> Transfer Fcn1/1
  Demux/3 -> Transfer Fcn2/1
  Transfer Fcn3/1 -> Mux/1
  Transfer Fcn1/1 -> Mux/2
  Transfer Fcn2/1 -> Mux/3

== system quadSimulationEnvironment/theta_comp/3vec_comp ==
  des : Inport
  meas : Inport  Port=2
  Demux1 : Demux  Outputs=3
  Demux2 : Demux  Outputs=3
  Mux2 : Mux  Inputs=2
  Mux3 : Mux  Inputs=2
  Mux4 : Mux  Inputs=2
  comp_x : Outport
  comp_y : Outport  Port=2
  comp_z : Outport  Port=3
  wires:
  Demux1/1 -> Mux2/1
  Demux1/2 -> Mux3/1
  Demux1/3 -> Mux4/1
  Demux2/1 -> Mux2/2
  Demux2/2 -> Mux3/2
  Demux2/3 -> Mux4/2
  Mux2/1 -> comp_x/1
  Mux3/1 -> comp_y/1
  Mux4/1 -> comp_z/1
  des/1 -> Demux1/1
  meas/1 -> Demux2/1

== system quadSimulationEnvironment/Outer control/position control/F(s) ==
  r_des : Inport
  Demux : Demux  Outputs=3
  Mux : Mux  Inputs=3
  m : TransferFcn  Numerator=[1/wf_z1 1]  Denominator=[1/wf_p1 1]
  m1 : TransferFcn  Numerator=[1/wf_z1 1]  Denominator=[1/wf_p1 1]
  m2 : TransferFcn  Numerator=[1/wf_z2 1]  Denominator=[1/wf_p2 1]
  m3 : TransferFcn  Numerator=[1/wf_z2 1]  Denominator=[1/wf_p2 1]
  m4 : TransferFcn  Numerator=[1/wf_z1 1]  Denominator=[1/wf_p1 1]
  m5 : TransferFcn  Numerator=[1/wf_z2 1]  Denominator=[1/wf_p2 1]
  r_des' : Outport
  wires:
  r_des/1 -> Demux/1
  Mux/1 -> r_des'/1
  Demux/1 -> m/1
  Demux/2 -> m1/1
  Demux/3 -> m4/1
  m/1 -> m3/1
  m3/1 -> Mux/1
  m1/1 -> m2/1
  m4/1 -> m5/1
  m2/1 -> Mux/2
  m5/1 -> Mux/3

== system quadSimulationEnvironment/Outer control/position control/double deriv ==
  u : Inport
  Demux : Demux  Outputs=3
  Mux : Mux  Inputs=3
  Transfer Fcn{1..6} (6 alike) : TransferFcn  Numerator=[1 0]  Denominator=[1/w_der 1]
  ddu' : Outport
  wires:
  u/1 -> Demux/1
  Demux/1 -> Transfer Fcn3/1
  Demux/2 -> Transfer Fcn2/1
  Demux/3 -> Transfer Fcn5/1
  Mux/1 -> ddu'/1
  Transfer Fcn3/1 -> Transfer Fcn1/1
  Transfer Fcn5/1 -> Transfer Fcn6/1
  Transfer Fcn1/1 -> Mux/1
  Transfer Fcn2/1 -> Transfer Fcn4/1
  Transfer Fcn6/1 -> Mux/3
  Transfer Fcn4/1 -> Mux/2

== system quadSimulationEnvironment/Outer control/position control/plantInverse ==
  r_des : Inport
  Demux : Demux  Outputs=3
  Gain : Gain  Gain=wmr^2/wt^2
  Mux : Mux  Inputs=3
  Transfer Fcn4 : TransferFcn  Commented=on  Numerator=[1/500 1]  Denominator=[1/750 1]
  m : TransferFcn  Numerator=[1 2*zt*wt wt^2]  Denominator=[1 2*zmr*wmr wmr^2]
  m1 : TransferFcn  Numerator=[1 2*zt*wt wt^2]  Denominator=[1 2*zmr*wmr wmr^2]
  m2 : TransferFcn  Numerator=[1 2*zt*wt wt^2]  Denominator=[1 2*zmr*wmr wmr^2]
  r_des' : Outport
  wires:
  r_des/1 -> Gain/1
  Gain/1 -> Demux/1
  m/1 -> Mux/1
  m1/1 -> Mux/2
  m2/1 -> Mux/3
  Demux/1 -> m/1
  Demux/2 -> m1/1
  Demux/3 -> m2/1
  Mux/1 -> r_des'/1

== matlab function quadSimulationEnvironment/Input mapping/yawFreeSig ==
  data: u input; sig_des output
function sig_des = fcn(u)

a = 4e-3;
% b = 3.0e-8;
l = 0.185;
dBand = 275;
dBand_mini = 60;

%% input to servo command
u1 = u(1);
u2 = u(2);
u3 = u(3);
% u4 = u(4);

sig_des = [ (l^2*u1^2 - 2*l*u1*u3 + u2^2 - u3^2)/(4*a*l^2*u1);
            (l^2*u1^2 - 2*l*u1*u2 - u2^2 + u3^2)/(4*a*l^2*u1);
            (l^2*u1^2 + 2*l*u1*u3 + u2^2 - u3^2)/(4*a*l^2*u1);
            (l^2*u1^2 + 2*l*u1*u2 - u2^2 + u3^2)/(4*a*l^2*u1)];
      
%% deadband offsetting         
for i=1:4
    if( sig_des(i) > dBand_mini )
        sig_des(i) = sig_des(i) + dBand;
    elseif( sig_des(i) < -dBand_mini )
        sig_des(i) = sig_des(i) - dBand;
    else
        sig_des(i) = 0;
    end
end

== matlab function quadSimulationEnvironment/Thrust vectoring/MATLAB Function ==
  data: u input; y output
function y = norm_u(u)

y = norm(u);

== matlab function quadSimulationEnvironment/Input mapping/mixing ==
  data: u0 input; sig_des output; u1 input; u2 input; u3 input; dw input
function sig_des = U2sig_des(u0,u1,u2,u3,dw)

MOTORSPEEDCONTROL_W0 = 780;
PWM_SIG0 = 525;
l = 0.19; 	
a =  3.5e-3;
b =  2.4375e-08;
dBand = 275;
dBand_mini = 60;
k1 = a;
k2 = 2*a/MOTORSPEEDCONTROL_W0*PWM_SIG0;
c1 = 2*b*PWM_SIG0;
c2 = 1*(b/MOTORSPEEDCONTROL_W0)*PWM_SIG0^2;

sig_des = [0 0 0 0]';
sig_des(1) = -(2*c1*u2 - c1*l*u0 - k1*l*u3 + 2*dw*c2*k1*l)/(4*c1*k1*l);
sig_des(2) = -(2*c1*u1 - c1*l*u0 + k1*l*u3 - 2*dw*c2*k1*l)/(4*c1*k1*l);
sig_des(3) =  (2*c1*u2 + c1*l*u0 + k1*l*u3 - 2*dw*c2*k1*l)/(4*c1*k1*l);
sig_des(4) =  (2*c1*u1 + c1*l*u0 - k1*l*u3 + 2*dw*c2*k1*l)/(4*c1*k1*l);

%% deadband offsetting         
for i=1:4
    if( sig_des(i) > dBand_mini )
        sig_des(i) = sig_des(i) + dBand;
    elseif( sig_des(i) < -dBand_mini )
        sig_des(i) = sig_des(i) - dBand;
    else
        sig_des(i) = 0;
    end
end

== matlab function quadSimulationEnvironment/Scopes/.1 ==
  data: x input; R_i output; dR_i output; Omega_b output; eta output; q output; zi output
function [R_i,dR_i,Omega_b,eta, q,zi] = out(x)
    coder.extrinsic('quat2angle','quat2dcm');
	R_i = x(1:3);
    dR_i = x(4:6);
    %Omega_b = 180/pi * X(7:9);
    Omega_b = x(11:13);
    q = quatnormalize([x(7) x(8) x(9) x(10)]);
    %neta = [0 0 0];
    %T = X(14);
    eta = [ 0 0 0 ];
    [eta(3) eta(2) eta(1)] = quat2angle(q,'ZYX');
    
    R = quat2dcm(q);
    zi = [0 0 0]';
    zi = R\[0 0 1]';
   % neta = 180/pi * neta;

== matlab function quadSimulationEnvironment/Input mapping/input2sig_des  ==
  data: u input; f_des output
function f_des = fcn(u)
%% parameters
l = 0.2;
c = 3.5e-3;
%% Torque to desired blade angle mapping      
u1 = u(1); u2 = u(2); u3 = u(3); u4 = u(4);

if( u1 ~= 0)
    f_des = 1/(4*c*l^2*u1)*[ c*l^2*u1^2+2*l^2*u4-2*c*l*u1*u3+c*u2^2-c*u3^2;
                             c*l^2*u1^2-2*l^2*u4-2*c*l*u1*u2-c*u2^2+c*u3^2;
                             c*l^2*u1^2+2*l^2*u4+2*c*l*u1*u3+c*u2^2-c*u3^2;
                             c*l^2*u1^2-2*l^2*u4+2*c*l*u1*u2-c*u2^2+c*u3^2];
else
    f_des = [0 0 0 0].';
end

== matlab function quadSimulationEnvironment/Quadcopter dynamics/getDifferentialEqns ==
  data: sig input; w input; q input; ddr output; Omega input; dq output; dOmega output; Tz output; f output; Mb output
function [ddr,dq,dOmega,Tz,f,Mb] = getDifferentialEqns(sig,w,q,Omega)
%% initialisation
coder.extrinsic('quatrotate','quatmultiply','quatconj')

f   = zeros(4,1);
tau = zeros(4,1);
Fi  = zeros(3,1);
dq  = zeros(4,1);
%% parameters
wmo = 600;
%a = 3.5e-3;
a = 0.0013;
%b = [2.1 2.2 2.55 2.7]*10^(-8);
b = [2.1 2.2 2.55 2.7]*10^(-8);
% b = 2.5e-8;
m = 0.634;
g = 9.8;
l = 0.20;
J = [3e-3  0     0
     0     2.95e-3  0
     0     0     5.29e-3];
Jm = 3e-6;
Jr = 1.57e-6;
%% Force and torque calcuation
% A = [0 0 1;0 0 1;0  0 1; 0 0 1];
% B = [0 l 0;l 0 0;0 -l 0;-l 0 0];
%     v = A*x(4:6) + B*omega_b;
v = zeros(4,1);
% sigo = [.1 .4 -.2 -.3]*pi/180/1.33e-4;
sigo = 0*1475*ones(1,4);

f(1) = forceEstimate(sig(1)+sigo(1),v(1),w(1));
f(2) = forceEstimate(sig(2)+sigo(2),v(2),w(2));
f(3) = forceEstimate(sig(3)+sigo(3),v(3),w(3));
f(4) = forceEstimate(sig(4)+sigo(4),v(4),w(4));
%f(1) = a*sig(1);
%f(2) = a*sig(2);
%f(3) = a*sig(3);
%f(4) = a*sig(4);

tau(1) =  torqueEstimate(sig(1)+sigo(1),v(1),w(1));
tau(2) = -torqueEstimate(sig(2)+sigo(2),v(2),w(2));
tau(3) =  torqueEstimate(sig(3)+sigo(3),v(3),w(3));
tau(4) = -torqueEstimate(sig(4)+sigo(4),v(4),w(4));

%tau(1) =  (b(1)/wmo^2)*wm(1)^2*( sig(1)+sigo(1) )^2;
%tau(2) = -(b(2)/wmo^2)*wm(2)^2*( sig(2)+sigo(2) )^2;
%tau(3) =  (b(3)/wmo^2)*wm(3)^2*( sig(3)+sigo(3) )^2;
%tau(4) = -(b(4)/wmo^2)*wm(4)^2*( sig(4)+sigo(4) )^2;
% tau(1) =  b(1)*sig(1)^2;
% tau(2) = -b(1)*sig(2)^2;
% tau(3) =  b(1)*sig(3)^2;
% tau(4) = -b(1)*sig(4)^2;

Tz = sum(f);
Fb = [0 0 Tz]';    
Mz = sum(tau);
%% Quaternion rate
dq = 1/2 * quatmultiply(q', [0 Omega'])';
%% Translational acceleration
G = [0 0 -m*g]';
Fi = quatrotate(quatconj(q'),Fb')';

ddr = 1/m*( Fi + G);
%% Rotational acceleration
Mb = [l*(f(4)-f(2));
      l*(f(3)-f(1));
            Mz    ];
mom_mr = [0 0 2*Jr*(w(1)-w(2))+Jm*(w(1)-w(2))]';
tau_gyro = cross(Omega,mom_mr);
%tau_gyro = 0;
dOmega = J \ ( Mb - cross(Omega,J*Omega) - tau_gyro );
%dw(3) = 0;
% dw = J\Mb;

== matlab function quadSimulationEnvironment/theta_comp/getRotVec ==
  data: q input; theta output
function theta = getRotationVector(q)

%% get rotation vector
alpha = 2*acos(q(1));
if( alpha ~= 0 )
    theta = q(2:4)*( alpha/sin(alpha/2) )';
else
    theta = [0 0 0]';
end

== matlab function quadSimulationEnvironment/theta_comp/getRotVec1 ==
  data: q input; theta output
function theta = getRotationVector(q)

%% get rotation vector
alpha = 2*acos(q(1));
if( alpha ~= 0 )
    theta = q(2:4)*( alpha/sin(alpha/2) )';
else
    theta = [0 0 0]';
end

== matlab function quadSimulationEnvironment/inner ref/getQuat ==
  data: q output; theta input
function q = getQuaternion(theta)

%% get quaternion
alpha = norm(theta);
if( alpha == 0 )
    q = [1 0 0 0]';
else
    q = [ cos(alpha/2) (sin(alpha/2)/alpha)*theta' ]';
end
